simulink subsystem "environment"  (R2023b)
settings: Solver=VariableStepAuto  StartTime=0.0  StopTime=10.0  RelTol=1e-3
libraries: nesl_utility x2, fl_lib x1, aerolibatmos2 x1
settings Model: Creator=imyrsini  LastModifiedBy=kroblet

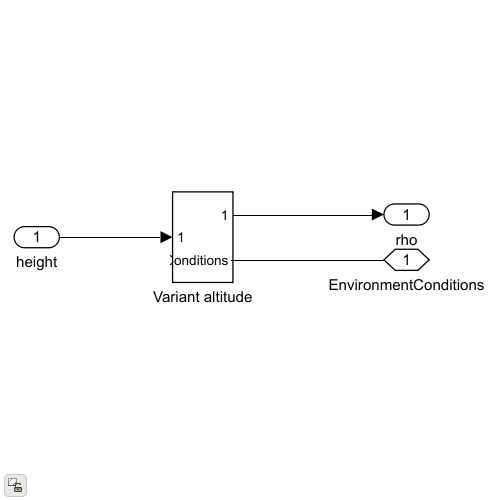
[thumbnail: Simulink's stored preview of the top-level diagram]
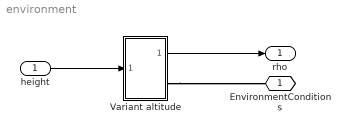
== system environment ==
  height : Inport
  Variant altitude : Subsystem  VariantControl=Choice_1
  EnvironmentConditions : PMIOPort  Side=Right
  rho : Outport
  wires:
  height/1 -> Variant altitude/1(Inport)
  Variant altitude/1(Outport) -> rho/1
  connections:
  Variant altitude/RConn1 -- EnvironmentConditions/RConn1

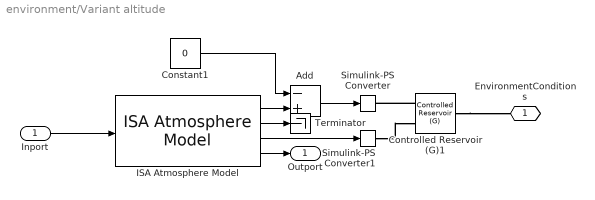
== system environment/Variant altitude ==
  Inport : Inport
  Add : Sum  Inputs=-+
  Constant1 : Constant  Value=0
  Controlled Reservoir (G)1 : fl_lib/Gas/Elements/Controlled Reservoir (G)  area_A=coreArea m^2
      settings: InternalSimscapePortConfiguration="{\"Bottom\":[],\"Left\":[{\"id\":\"A\",\"label\":\"A\",\"type\":\"foundation.gas.gas\"}],\"Right\":[{\"id\":\"T_in\",\"label\":\"T\",\"type\":\"input\"},{\"id\":\"p_in\",\"label\":\"P\",\"type\":\"input\"}],\"Top\":[]}"
  ISA Atmosphere Model : aerolibatmos2/ISA Atmosphere Model  useExtended=off  action=Warning  custom=off  viscosityOut=off  g=9.80665  gamma=1.4  R=287.0531  L=0.0065  h_trop=11000  h_strat=20000  rho0=1.225  P0=101325  T0=288.15  h0=0
  Simulink-PS Converter : nesl_utility/Simulink-PS Converter  PhysicalDomain=network_engine_domain  SubClassName=ps_input  LeftPortType=input  RightPortType=output  PseudoPeriodic=off  Frequencies=[]  NoiseDistribution=none  NoiseParameters=[]  Unit=K  AffineConversion=off  FilteringAndDerivatives=provide  SimscapeFilterOrder=1  InputFilterTimeConstant=0.001  UdotUserProvided=0
  Simulink-PS Converter1 : nesl_utility/Simulink-PS Converter  PhysicalDomain=network_engine_domain  SubClassName=ps_input  LeftPortType=input  RightPortType=output  PseudoPeriodic=off  Frequencies=[]  NoiseDistribution=none  NoiseParameters=[]  Unit=Pa  AffineConversion=off  FilteringAndDerivatives=provide  SimscapeFilterOrder=1  InputFilterTimeConstant=0.001  UdotUserProvided=0
  Terminator : Terminator
  EnvironmentConditions : PMIOPort  Side=Right
  Outport : Outport
  wires:
  ISA Atmosphere Model/3 -> Simulink-PS Converter1/1
  ISA Atmosphere Model/2 -> Terminator/1
  Inport/1 -> ISA Atmosphere Model/1
  Constant1/1 -> Add/1
  ISA Atmosphere Model/4 -> Outport/1
  ISA Atmosphere Model/1 -> Add/2
  Add/1 -> Simulink-PS Converter/1
  connections:
  Controlled Reservoir (G)1/LConn1 -- EnvironmentConditions/RConn1
  Controlled Reservoir (G)1/RConn1 -- Simulink-PS Converter/RConn1
  Simulink-PS Converter1/RConn1 -- Controlled Reservoir (G)1/RConn2
